simulink model "FLWSimNoise"  (R2017b)
settings: Solver=ode45  StartTime=0.0  StopTime=12  MaxStep=0.001  RelTol=1e-3
InitFcn:
  | SimInit
  | CustomInit
values from neighbouring files (symbols this model uses):
  externalForce = -3000    [main.m]    (also in sim_pert.m = 1100)
undefined symbols (not defined in the file or in its folder): IC, info
libraries: simulink x5, commchan3 x2
settings Model: Creator=81068  LastModifiedBy=mungam
settings SFSimCC: SimUserSources=|
  | CoriolisTerm_src.c
  | GravityVector_src.c
  | InertiaMatrix_src.c
  | 
  | AMBody_LeftShin_src.c
  | AMBody_LeftThigh_src.c
  | AMBody_RightShin_src.c
  | AMBody_RightThigh_src.c
  | AMBody_torso_src.c
  | AMWorld_LeftShin_src.c
  | AMWorld_LeftThigh_src.c
  | AMWorld_RightShin_src.c
  | AMWorld_RightThigh_src.c
  | AMWorld_torso_src.c
  | dJb_Head_src.c
  | dJb_LeftHip_src.c
  | dJb_LeftKnee_src.c
  | dJb_LeftShin_src.c
  | dJb_LeftThigh_src.c
  | dJb_LeftToe_src.c
  | dJb_RightHip_src.c
  | dJb_RightKnee_src.c
  | dJb_RightShin_src.c
  | dJb_RightThigh_src.c
  | dJb_RightToe_src.c
  | dJb_torso_src.c
  | dJp_COM_src.c
  | dJp_Head_src.c
  | dJp_LeftHip_src.c
  | dJp_LeftKnee_src.c
  | dJp_LeftShin_src.c
  | dJp_LeftThigh_src.c
  | dJp_LeftToe_src.c
  | dJp_RightHip_src.c
  | dJp_RightKnee_src.c
  | dJp_RightShin_src.c
  | dJp_RightThigh_src.c
  | dJp_RightToe_src.c
  | dJp_torso_src.c
  | dJs_Head_src.c
  | dJs_LeftHip_src.c
  | dJs_LeftKnee_src.c
  | dJs_LeftShin_src.c
  | dJs_LeftThigh_src.c
  | dJs_LeftToe_src.c
  | dJs_RightHip_src.c
  | dJs_RightKnee_src.c
  | dJs_RightShin_src.c
  | dJs_RightThigh_src.c
  | dJs_RightToe_src.c
  | dJs_torso_src.c
  | dR_Head_src.c
  | dR_LeftHip_src.c
  | dR_LeftKnee_src.c
  | dR_LeftShin_src.c
  | dR_LeftThigh_src.c
  | dR_LeftToe_src.c
  | dR_RightHip_src.c
  | dR_RightKnee_src.c
  | dR_RightShin_src.c
  | dR_RightThigh_src.c
  | dR_RightToe_src.c
  | dR_torso_src.c
  | dT_Head_src.c
  | dT_LeftHip_src.c
  | dT_LeftKnee_src.c
  | dT_LeftShin_src.c
  | dT_LeftThigh_src.c
  | dT_LeftToe_src.c
  | dT_RightHip_src.c
  | dT_RightKnee_src.c
  | dT_RightShin_src.c
  | dT_RightThigh_src.c
  | dT_RightToe_src.c
  | dT_torso_src.c
  | Inertia_LeftShin_src.c
  | Inertia_LeftThigh_src.c
  | Inertia_RightShin_src.c
  | Inertia_RightThigh_src.c
  | Inertia_torso_src.c
  | Jb_Head_src.c
  | Jb_LeftHip_src.c
  | Jb_LeftKnee_src.c
  | Jb_LeftShin_src.c
  | Jb_LeftThigh_src.c
  | Jb_LeftToe_src.c
  | Jb_RightHip_src.c
  | Jb_RightKnee_src.c
  | Jb_RightShin_src.c
  | Jb_RightThigh_src.c
  | Jb_RightToe_src.c
  | Jb_torso_src.c
  | Jp_COM_src.c
  | Jp_Head_src.c
  | Jp_LeftHip_src.c
  | Jp_LeftKnee_src.c
  | Jp_LeftShin_src.c
  | Jp_LeftThigh_src.c
  | Jp_LeftToe_src.c
  | Jp_RightHip_src.c
  | Jp_RightKnee_src.c
  | Jp_RightShin_src.c
  | Jp_RightThigh_src.c
  | Jp_RightToe_src.c
  | Jp_torso_src.c
  | Js_Head_src.c
  | Js_LeftHip_src.c
  | Js_LeftKnee_src.c
  | Js_LeftShin_src.c
  | Js_LeftThigh_src.c
  | Js_LeftToe_src.c
  | Js_RightHip_src.c
  | Js_RightKnee_src.c
  | Js_RightShin_src.c
  | Js_RightThigh_src.c
  | Js_RightToe_src.c
  | Js_torso_src.c
  | p_COM_src.c
  | p_Head_src.c
  | p_LeftHip_src.c
  | p_LeftKnee_src.c
  | p_LeftShin_src.c
  | p_LeftThigh_src.c
  | p_LeftToe_src.c
  | p_RightHip_src.c
  | p_RightKnee_src.c
  | p_RightShin_src.c
  | p_RightThigh_src.c
  | p_RightToe_src.c
  | p_torso_src.c
  | R_Head_src.c
  | R_LeftHip_src.c
  | R_LeftKnee_src.c
  | R_LeftShin_src.c
  | R_LeftThigh_src.c
  | R_LeftToe_src.c
  | R_RightHip_src.c
  | R_RightKnee_src.c
  | R_RightShin_src.c
  | R_RightThigh_src.c
  | R_RightToe_src.c
  | R_torso_src.c
  | T_Head_src.c
  | T_LeftHip_src.c
  | T_LeftKnee_src.c
  | T_LeftShin_src.c
  | T_LeftThigh_src.c
  | T_LeftToe_src.c
  | T_RightHip_src.c
  | T_RightKnee_src.c
  | T_RightShin_src.c
  | T_RightThigh_src.c
  | T_RightToe_src.c
  | T_torso_src.c
settings SFSimCC: SimUserIncludeDirs=|
  | D:\Dropbox (DynamicLegLocomotion)\robots\codes\SimpleModels\FiveLinkWalker\Simulation\Model\dyn\src
  | D:\Dropbox (DynamicLegLocomotion)\robots\codes\SimpleModels\FiveLinkWalker\Simulation\Model\kin\src
settings CodeAppCC: StateflowObjectComments=on

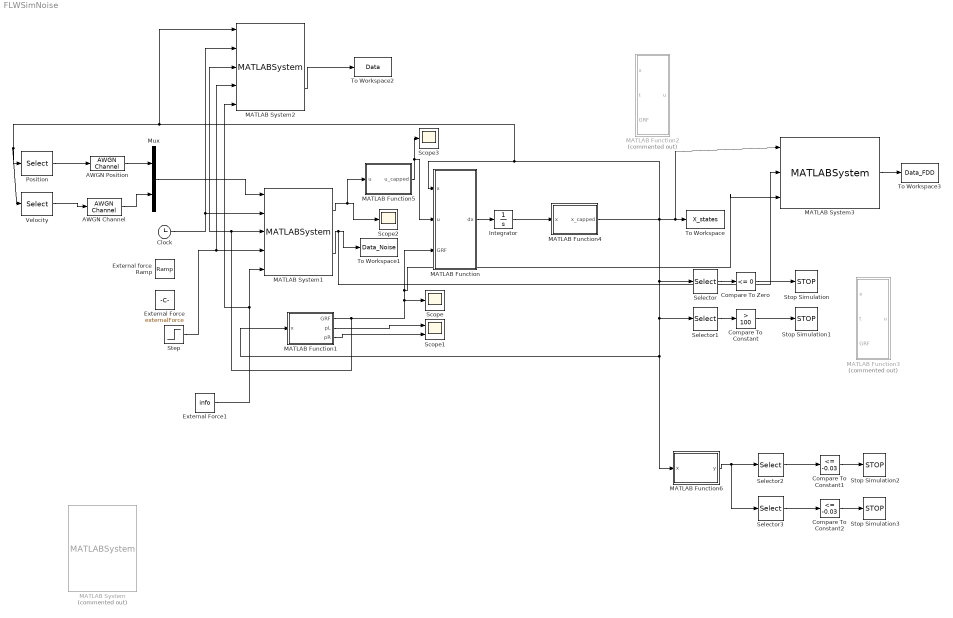
== system FLWSimNoise ==
  AWGN Channel : commchan3/AWGN Channel  InputProcessing=Columns as channels (frame based)  seed=4  noiseMode=Variance from mask  EbNodB=10  EsNodB=10  SNRdB=10  bitsPerSym=1  Ps=1  Tsym=1  variance=cov_dq
  AWGN Position : commchan3/AWGN Channel  InputProcessing=Columns as channels (frame based)  seed=3  noiseMode=Variance from mask  EbNodB=10  EsNodB=10  SNRdB=10  bitsPerSym=1  Ps=1  Tsym=1  variance=cov_q
  Clock : Clock
  Compare To Constant : simulink/Logic and Bit Operations/Compare To Constant  relop=>  const=100  OutDataTypeStr=boolean
  Compare To Constant1 : simulink/Logic and Bit Operations/Compare To Constant  relop=<=  const=-0.03  OutDataTypeStr=boolean
  Compare To Constant2 : simulink/Logic and Bit Operations/Compare To Constant  relop=<=  const=-0.03  OutDataTypeStr=boolean
  Compare To Zero : simulink/Logic and Bit Operations/Compare To Zero  relop=<=  OutDataTypeStr=boolean
  External Force : Constant  Value=externalForce
  External Force1 : Constant  Value=info  OutDataTypeStr=Bus: info_bus
  External force Ramp : simulink/Sources/Ramp  slope=250  start=0  X0=0
  Integrator : Integrator  InitialCondition=IC
  MATLAB Function : MATLAB Function  TreatAsAtomicUnit=on
  MATLAB Function1 : MATLAB Function  TreatAsAtomicUnit=on
  MATLAB Function2 : MATLAB Function  Commented=on  TreatAsAtomicUnit=on
  MATLAB Function3 : MATLAB Function  Commented=on  TreatAsAtomicUnit=on
  MATLAB Function4 : MATLAB Function  TreatAsAtomicUnit=on
  MATLAB Function5 : MATLAB Function  TreatAsAtomicUnit=on
  MATLAB Function6 : MATLAB Function  TreatAsAtomicUnit=on
  MATLAB System : MATLABSystem  Commented=on  System=FLW_Controller_1  SimulateUsing=Code generation
      mask Type: FLW_Controller_1
      mask Display:
      | disp('FLW_Controller_1');
      | port_label('input',1,'x');
      | port_label('input',2,'t');
      | port_label('input',3,'GRF');
      | port_label('output',1,'u');
      | port_label('output',2,'Data');
  MATLAB System1 : MATLABSystem  System=FLW_Controller_2  SimulateUsing=Interpreted execution
      mask Type: FLW_Controller_2
      mask Display:
      | disp('FLW_Controller_2');
      | port_label('input',1,'x');
      | port_label('input',2,'t');
      | port_label('input',3,'GRF');
      | port_label('input',4,'External Force');
      | port_label('input',5,'info');
      | port_label('output',1,'u');
      | port_label('output',2,'Data');
  MATLAB System2 : MATLABSystem  System=FLW_Controller_2  SimulateUsing=Interpreted execution
      mask Type: FLW_Controller_2
      mask Display:
      | disp('FLW_Controller_2');
      | port_label('input',1,'x');
      | port_label('input',2,'t');
      | port_label('input',3,'GRF');
      | port_label('input',4,'External Force');
      | port_label('input',5,'info');
      | port_label('output',1,'u');
      | port_label('output',2,'Data');
  MATLAB System3 : MATLABSystem  System=FDD_Data_Plant  SimulateUsing=Interpreted execution
      mask Type: FDD_Data_Plant
      mask Display:
      | disp('FDD_Data_Plant');
      | port_label('input',1,'x');
      | port_label('input',2,'ctrl_info');
      | port_label('input',3,'GRF');
      | port_label('output',1,'Data');
  Mux : Mux  Inputs=2
  Position : Selector  InputPortWidth=14  IndexOptions=Index vector (dialog)  Indices=[1:7]  OutputSizes=1
  Scope : Scope
  Scope1 : Scope  NumInputPorts=2
  Scope2 : Scope
  Scope3 : Scope
  Selector : Selector  InputPortWidth=14  IndexOptions=Index vector (dialog)  Indices=[2]  OutputSizes=1
  Selector1 : Selector  InputPortWidth=14  IndexOptions=Index vector (dialog)  Indices=[8]  OutputSizes=1
  Selector2 : Selector  InputPortWidth=6  IndexOptions=Index vector (dialog)  Indices=[3]  OutputSizes=1
  Selector3 : Selector  InputPortWidth=6  IndexOptions=Index vector (dialog)  Indices=[6]  OutputSizes=1
  Step : Step  Time=5  After=externalForce  SampleTime=0
  Stop Simulation{,1..3} (4 alike) : Stop
  To Workspace : ToWorkspace  VariableName=X_states  SampleTime=-1
  To Workspace1 : ToWorkspace  VariableName=Data_Noise  SaveFormat=Timeseries  SampleTime=-1
  To Workspace2 : ToWorkspace  VariableName=Data  SaveFormat=Timeseries  SampleTime=-1
  To Workspace3 : ToWorkspace  VariableName=Data_FDD  SaveFormat=Timeseries  SampleTime=-1
  Velocity : Selector  InputPortWidth=14  IndexOptions=Index vector (dialog)  Indices=[8:14]  OutputSizes=1
  wires:
  MATLAB Function/1(dx) -> Integrator/1
  MATLAB Function1/1(GRF) -> MATLAB System1/3, MATLAB System2/3, Scope/1, MATLAB System3/3, MATLAB Function/3(GRF)
  Integrator/1 -> MATLAB Function4/1(x)
  MATLAB System1/1 -> MATLAB Function5/1(u), Scope2/1
  MATLAB Function1/2(pL) -> Scope1/1
  Selector/1 -> Compare To Zero/1
  Clock/1 -> MATLAB System1/2, MATLAB System2/2
  MATLAB System1/2 -> MATLAB System3/2, To Workspace1/1
  Selector1/1 -> Compare To Constant/1
  MATLAB Function1/3(pR) -> Scope1/2
  MATLAB Function4/1(x_capped) -> MATLAB Function1/1(x), MATLAB Function6/1(x), Selector1/1, Selector/1, MATLAB System2/1, Velocity/1, Position/1, MATLAB Function/1(x), MATLAB System3/1, To Workspace/1
  Compare To Constant/1 -> Stop Simulation1/1
  Compare To Zero/1 -> Stop Simulation/1
  MATLAB Function5/1(u_capped) -> MATLAB Function/2(u), Scope3/1
  Position/1 -> AWGN Position/1
  AWGN Position/1 -> Mux/1
  AWGN Channel/1 -> Mux/2
  Mux/1 -> MATLAB System1/1
  Velocity/1 -> AWGN Channel/1
  External Force1/1 -> MATLAB System2/5, MATLAB System1/5
  MATLAB System2/2 -> To Workspace2/1
  MATLAB Function6/1(y) -> Selector3/1, Selector2/1
  Selector2/1 -> Compare To Constant1/1
  Compare To Constant1/1 -> Stop Simulation2/1
  Selector3/1 -> Compare To Constant2/1
  Compare To Constant2/1 -> Stop Simulation3/1
  MATLAB System3/1 -> To Workspace3/1
  Step/1 -> MATLAB System2/4, MATLAB System1/4

== matlab function FLWSimNoise/MATLAB Function1 ==
  data: x input; GRF output; pL output; pR output
function [GRF,pL,pR] = fcn(x)
stiffness_v = 60000;
damping_v = 1000;
damping_h = 10000;
FC = 10; % Friction Cone
q = x(1:7);
dq = x(8:14);
GRF= zeros(6,1);

pL = p_LeftToe(q);
pR = p_RightToe(q);
vL = Jp_LeftToe(q)*dq;
vR = Jp_RightToe(q)*dq;



if pL(3)<0
    GRF_Lx = -damping_h*vL(1);
    GRF_Lz = -stiffness_v*pL(3)-damping_v*vL(3);
    GRF(1) = GRF_Lx;
    GRF(3) = GRF_Lz;
end

if pR(3)<0
    GRF_Rx = -damping_h*vR(1);
    GRF_Rz = -stiffness_v*pR(3)-damping_v*vR(3);
    GRF(4) = GRF_Rx;
    GRF(6) = GRF_Rz;
end

GRF(3) = max([0,GRF(3)]);
GRF(6) = max([0,GRF(6)]);

GRF(1) = median([GRF(1), FC*GRF(3), - FC*GRF(3)]);
GRF(4) = median([GRF(4), FC*GRF(6), - FC*GRF(6)]);
end

== matlab function FLWSimNoise/MATLAB Function ==
  data: x input; u input; dx output; GRF input
function dx = ContinuousModel(x,u,GRF)
dx = zeros(size(x));
q = x(1:7);
dq = x(8:end);

M = InertiaMatrix(q);
C = CoriolisTerm(q,dq);
G = GravityVector(q);
B = [zeros(3,4);eye(4)];

JgL = Jp_LeftToe(q);
JgR = Jp_RightToe(q);
Jg = [JgL;JgR];

ddq = M^-1*(-C-G+B*u+Jg'*GRF);

dx = [dq;ddq];

end

== matlab function FLWSimNoise/MATLAB Function2 ==
  data: x input; u output; t input; GRF input
function u = walk_in_place(x,t,GRF)
q = x(1:7);
dq = x(8:14);
% Let the output be torso angle, hip height and x,z of swing feet.
T = 0.4; % walking period
Kd = 50;
Kp = 400;
s = rem(t,T)/T;
ds = 1/T;

if mod(fix(t/T),2)
    stanceLeg = 1;
else
    stanceLeg = -1;
end
    


hr= [-pi/6;0.6;0;(s-0.5)^2+0.35];
dhr = [0;0;0;2*(s-0.5)*ds];
ddhr = [0;0;0;2*ds^2];

p_LT = p_LeftToe(q);
p_RT = p_RightToe(q);
Jp_LT = Jp_LeftToe(q);
Jp_RT = Jp_RightToe(q);
dJp_LT = dJp_LeftToe(q,dq);
dJp_RT = dJp_RightToe(q,dq);

% r means relative position to hip
J_basexyz = zeros(3,7); J_basexyz(1,1) = 1; J_basexyz(3,2) = 1; 
rp_LT = [q(1);0;q(2)] - p_LeftToe(q);
rp_RT = [q(1);0;q(2)] - p_RightToe(q);
Jrp_LT = J_basexyz - Jp_LeftToe(q);
Jrp_RT = J_basexyz - Jp_RightToe(q);
dJrp_LT = -dJp_LeftToe(q,dq);
dJrp_RT = -dJp_RightToe(q,dq);

M = InertiaMatrix(q);
C = CoriolisTerm(q,dq);
G = GravityVector(q);
B = [zeros(3,4);eye(4)];

q1 = q;
q2 = q1; q2([4,5,6,7]) = q2([6,7,4,5]);
% q = q2;
if stanceLeg == -1
    % Jh is jacobian for output
    Jh = zeros(4,7);
    dJh = zeros(4,7);
    
    Jh(1,3) = 1;
    Jh(2,:) = Jrp_LT(3,:);
    Jh([3,4],:) = Jrp_RT([1,3],:);
    
    dJh(2,:) = dJrp_LT(3,:);
    dJh([3,4],:) = dJrp_RT([1,3],:);
    
    h0 = [q(3);rp_LT(3);rp_RT([1,3])];
    dh0 = Jh*dq;
    %Jg is Jacobian for ground constraint
    Jg = Jp_LT([1,3],:);
    dJg = dJp_LT([1,3],:);
    
else
    
    Jh = zeros(4,7);
    dJh = zeros(4,7);
    
    Jh(1,3) = 1;
    Jh(2,:) = Jrp_RT(3,:);
    Jh([3,4],:) = Jrp_LT([1,3],:);
    
    dJh(2,:) = dJrp_RT(3,:);
    dJh([3,4],:) = dJrp_LT([1,3],:);
    
    h0 = [q(3);rp_RT(3);rp_LT([1,3])];
    dh0 = Jh*dq;
    
    Jg = Jp_RT([1,3],:);
    dJg = dJp_RT([1,3],:);
    
end

Me = [M -Jg';Jg,zeros(2,2)];
He = [C+G;dJg*dq];
Be = [B;zeros(2,4)];

S = [eye(7),zeros(7,2)]; % S is used to seperate ddq with Fg;

y = h0 - hr;
dy = dh0 - dhr;

u = (Jh*S*Me^-1*Be)^-1*(-Kd*dy-Kp*y+ddhr+Jh*S*Me^-1*He);
end

== matlab function FLWSimNoise/MATLAB Function3 ==
  data: x input; u output; t input; GRF input
function u = controller(x,t,GRF)
q = x(1:7);
dq = x(8:14);
% Let the output be torso angle, com height and delta x,delta z of swing
% feet and com. delta = p_com - p_swfeet.
T = 0.4; % walking period
Kd = 50;
Kp = 400;
s = rem(t,T)/T;
ds = 1/T;

if mod(fix(t/T),2)==1 && GRF(6)>100
    stanceLeg = 1;
elseif mod(fix(t/T),2)==1 && GRF(6)<=100
    stanceLeg = -1;
elseif mod(fix(t/T),2) == 0 && GRF(3)<=100
    stanceLeg = -1;
else
    stanceLeg = 1;
end
    


hr= [-pi/6;0.6;0;(s-0.5)^2+0.35];
dhr = [0;0;0;2*(s-0.5)*ds];
ddhr = [0;0;0;2*ds^2];

p_LT = p_LeftToe(q);
p_RT = p_RightToe(q);
Jp_LT = Jp_LeftToe(q);
Jp_RT = Jp_RightToe(q);
dJp_LT = dJp_LeftToe(q,dq);
dJp_RT = dJp_RightToe(q,dq);

% r means relative position to com

rp_LT = p_COM(q) - p_LeftToe(q);
rp_RT = p_COM(q) - p_RightToe(q);
Jrp_LT = Jp_COM(q) - Jp_LeftToe(q);
Jrp_RT = Jp_COM(q) - Jp_RightToe(q);
dJrp_LT = dJp_COM(q,dq)-dJp_LeftToe(q,dq);
dJrp_RT = dJp_COM(q,dq)-dJp_RightToe(q,dq);

M = InertiaMatrix(q);
C = CoriolisTerm(q,dq);
G = GravityVector(q);
B = [zeros(3,4);eye(4)];

% q1 = q;
% q2 = q1; q2([4,5,6,7]) = q2([6,7,4,5]);
% %q = q2;
if stanceLeg == -1
    % Jh is jacobian for output
    Jh = zeros(4,7);
    dJh = zeros(4,7);
    
    Jh(1,3) = 1;
    Jh(2,:) = Jrp_LT(3,:);
    Jh([3,4],:) = Jrp_RT([1,3],:);
    
    dJh(2,:) = dJrp_LT(3,:);
    dJh([3,4],:) = dJrp_RT([1,3],:);
    
    h0 = [q(3);rp_LT(3);rp_RT([1,3])];
    dh0 = Jh*dq;
    %Jg is Jacobian for ground constraint
    Jg = Jp_LT([1,3],:);
    dJg = dJp_LT([1,3],:);
    
else
    
    Jh = zeros(4,7);
    dJh = zeros(4,7);
    
    Jh(1,3) = 1;
    Jh(2,:) = Jrp_RT(3,:);
    Jh([3,4],:) = Jrp_LT([1,3],:);
    
    dJh(2,:) = dJrp_RT(3,:);
    dJh([3,4],:) = dJrp_LT([1,3],:);
    
    h0 = [q(3);rp_RT(3);rp_LT([1,3])];
    dh0 = Jh*dq;
    
    Jg = Jp_RT([1,3],:);
    dJg = dJp_RT([1,3],:);
    
end

Me = [M -Jg';Jg,zeros(2,2)];
He = [C+G;dJg*dq];
Be = [B;zeros(2,4)];

S = [eye(7),zeros(7,2)]; % S is used to seperate ddq with Fg;

y = h0 - hr;
dy = dh0 - dhr;

u = (Jh*S*Me^-1*Be)^-1*(-Kd*dy-Kp*y+ddhr+Jh*S*Me^-1*He);
end

== matlab function FLWSimNoise/MATLAB Function4 ==
  data: x input; x_capped output
function x_capped = capStates(x)
%this function imposes the state limits for the rabbit model
q_lb = [-inf, 0.5, -1,-2, 0, -2, 0];
q_ub = [inf, 2, 1,  0.26, 2.1, 0.26, 2.1];
dq_lb = -20*ones(1,7);
dq_ub = 20*ones(1,7);
x_lb=[q_lb,dq_lb];
x_ub=[q_ub,dq_ub];
x_capped=x;
for i=1:length(x_capped)
    if x_capped(i) < x_lb(i) 
        x_capped(i)=x_lb(i);
    elseif x_capped(i) > x_ub(i)
        x_capped(i) = x_ub(i);
    end
end

== matlab function FLWSimNoise/MATLAB Function5 ==
  data: u input; u_capped output
function u_capped = capInputs(u)
u_capped=u;
lim=200;
for i=1:length(u)
    if u_capped(i) > lim
        u_capped(i) = lim;
    elseif u_capped(i) < -lim
        u_capped(i)=-lim;
    end
%     u_capped=zeros(size(u));
end

== matlab function FLWSimNoise/MATLAB Function6 ==
  data: x input; y output
function y  = ToePositions(x)
q=x(1:7);
p_LT = p_LeftToe(q);
p_RT = p_RightToe(q);

y = [p_LT;p_RT];


end
